simulink model "pmsm_vector_ctrl_osm_3_2021_06_21"  (R2020a)
settings: Solver=daessc  StartTime=0.0  StopTime=simlength  MaxStep=Ts/10
values from neighbouring files (symbols this model uses):
  dead_time = 0    [init_pmsm_2021_06_21.m]
  delayINV_modA = 0    [init_pmsm_2021_06_21.m]
  fPWM_INV = 8e3    (= 8000)    [init_pmsm_2021_06_21.m]
  Ibez = 450    [init_pmsm_2021_06_21.m]
  Jm = 1    [init_pmsm_2021_06_21.m]
  ki = 18    [init_pmsm_2021_06_21.m]
  kp = 2    [init_pmsm_2021_06_21.m]
  Ld = 1.7e-3    (= 0.0017)    [init_pmsm_2021_06_21.m]
  Lq = 4.3e-3    (= 0.0043)    [init_pmsm_2021_06_21.m]
  psi_m = 890/sqrt(3)/(3100/60*number_poles/2*2*pi)    [init_pmsm_2021_06_21.m]
  simlength = 5    [init_pmsm_2021_06_21.m]
  Tc = 1e-5    (= 1e-05)    [init_pmsm_2021_06_21.m]
  Ts = 1/10e3    (= 0.0001)    [init_pmsm_2021_06_21.m]
libraries: fl_lib x23, nesl_utility x22, ee_lib x6, flexshaft_lib x1, pmsm_uvw_lib x1
(part 2 of 2)

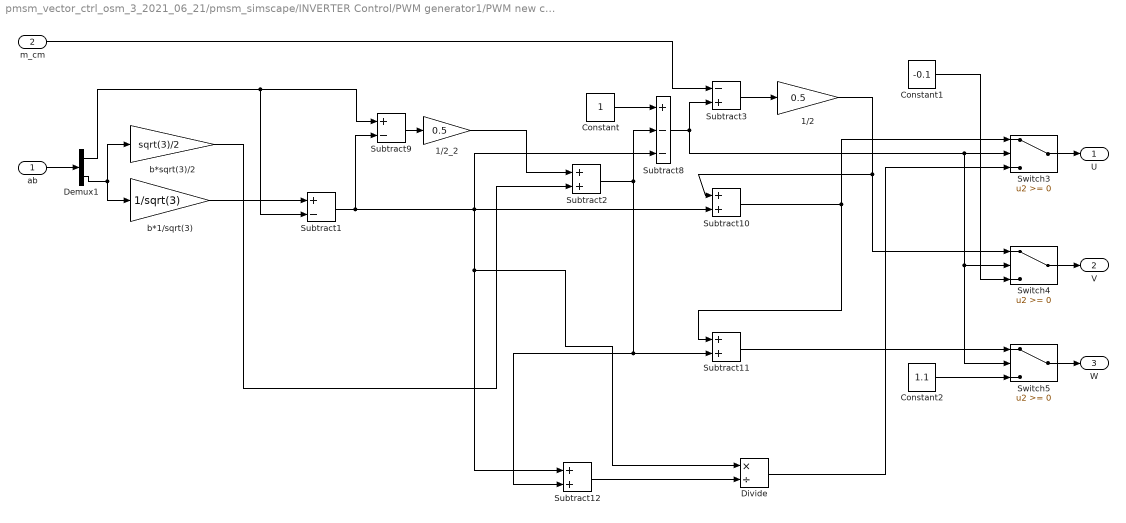
== system pmsm_vector_ctrl_osm_3_2021_06_21/pmsm_simscape/INVERTER Control/PWM generator1/PWM new cm modulation/Sector2 ==
  ab : Inport
  m_cm : Inport  Port=2
  1/2 : Gain  Gain=0.5
  1/2_2 : Gain  Gain=0.5
  Constant : Constant
  Constant1 : Constant  Value=-0.1
  Constant2 : Constant  Value=1.1
  Demux1 : Demux  Outputs=2
  Divide : Product  Inputs=*/
  Subtract1 : Sum  Inputs=+-
  Subtract{2,10..12} (4 alike) : Sum
  Subtract3 : Sum  Inputs=-+
  Subtract8 : Sum  Inputs=+--
  Subtract9 : Sum  Inputs=+-
  Switch3 : Switch
  Switch4 : Switch
  Switch5 : Switch
  b*1/sqrt(3) : Gain  Gain=1/sqrt(3)
  b*sqrt(3)/2 : Gain  Gain=sqrt(3)/2
  U : Outport
  V : Outport  Port=2
  W : Outport  Port=3
  wires:
  1/2/1 -> Switch4/1, Subtract10/1
  m_cm/1 -> Subtract3/1
  Subtract10/1 -> Subtract11/1, Switch3/1
  Constant2/1 -> Switch5/3
  Divide/1 -> Switch3/3
  Constant1/1 -> Switch4/3
  Subtract3/1 -> 1/2/1
  Subtract2/1 -> Subtract11/2, Subtract12/2, Subtract8/2
  b*sqrt(3)/2/1 -> Subtract2/2
  1/2_2/1 -> Subtract2/1
  Subtract9/1 -> 1/2_2/1
  Subtract1/1 -> Subtract9/2, Subtract8/3, Subtract10/2, Divide/1, Subtract12/1
  b*1/sqrt(3)/1 -> Subtract1/1
  Switch5/1 -> W/1
  Switch4/1 -> V/1
  Switch3/1 -> U/1
  ab/1 -> Demux1/1
  Subtract8/1 -> Switch5/2, Switch4/2, Switch3/2, Subtract3/2
  Constant/1 -> Subtract8/1
  Subtract11/1 -> Switch5/1
  Subtract12/1 -> Divide/2
  Demux1/1 -> Subtract1/2, Subtract9/1
  Demux1/2 -> b*sqrt(3)/2/1, b*1/sqrt(3)/1

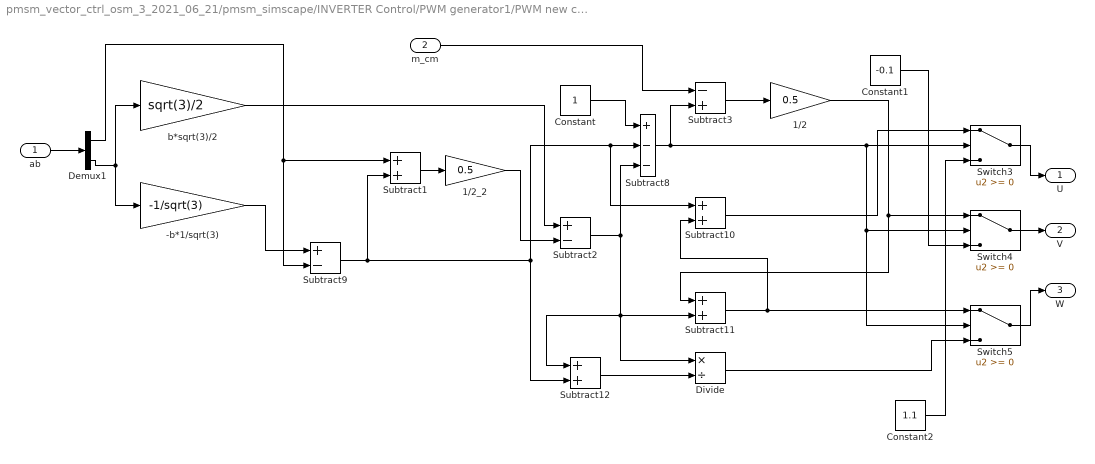
== system pmsm_vector_ctrl_osm_3_2021_06_21/pmsm_simscape/INVERTER Control/PWM generator1/PWM new cm modulation/Sector3 ==
  ab : Inport
  m_cm : Inport  Port=2
  -b*1/sqrt(3) : Gain  Gain=-1/sqrt(3)
  1/2 : Gain  Gain=0.5
  1/2_2 : Gain  Gain=0.5
  Constant : Constant
  Constant1 : Constant  Value=-0.1
  Constant2 : Constant  Value=1.1
  Demux1 : Demux  Outputs=2
  Divide : Product  Inputs=*/
  Subtract{1,10..12} (4 alike) : Sum
  Subtract2 : Sum  Inputs=+-
  Subtract3 : Sum  Inputs=-+
  Subtract8 : Sum  Inputs=+--
  Subtract9 : Sum  Inputs=+-
  Switch3 : Switch
  Switch4 : Switch
  Switch5 : Switch
  b*sqrt(3)/2 : Gain  Gain=sqrt(3)/2
  U : Outport
  V : Outport  Port=2
  W : Outport  Port=3
  wires:
  1/2/1 -> Switch4/1, Subtract11/1
  m_cm/1 -> Subtract3/1
  Constant1/1 -> Switch4/3
  Constant2/1 -> Switch3/3
  Divide/1 -> Switch5/3
  Subtract10/1 -> Switch3/1
  Subtract11/1 -> Subtract10/2, Switch5/1
  Subtract3/1 -> 1/2/1
  1/2_2/1 -> Subtract2/2
  Subtract1/1 -> 1/2_2/1
  b*sqrt(3)/2/1 -> Subtract2/1
  Subtract2/1 -> Subtract11/2, Divide/1, Subtract12/1, Subtract8/3
  Subtract9/1 -> Subtract12/2, Subtract8/2, Subtract10/1, Subtract1/2
  Demux1/1 -> Subtract9/2, Subtract1/1
  -b*1/sqrt(3)/1 -> Subtract9/1
  Demux1/2 -> -b*1/sqrt(3)/1, b*sqrt(3)/2/1
  Subtract12/1 -> Divide/2
  Constant/1 -> Subtract8/1
  Subtract8/1 -> Switch3/2, Switch4/2, Switch5/2, Subtract3/2
  ab/1 -> Demux1/1
  Switch3/1 -> U/1
  Switch4/1 -> V/1
  Switch5/1 -> W/1

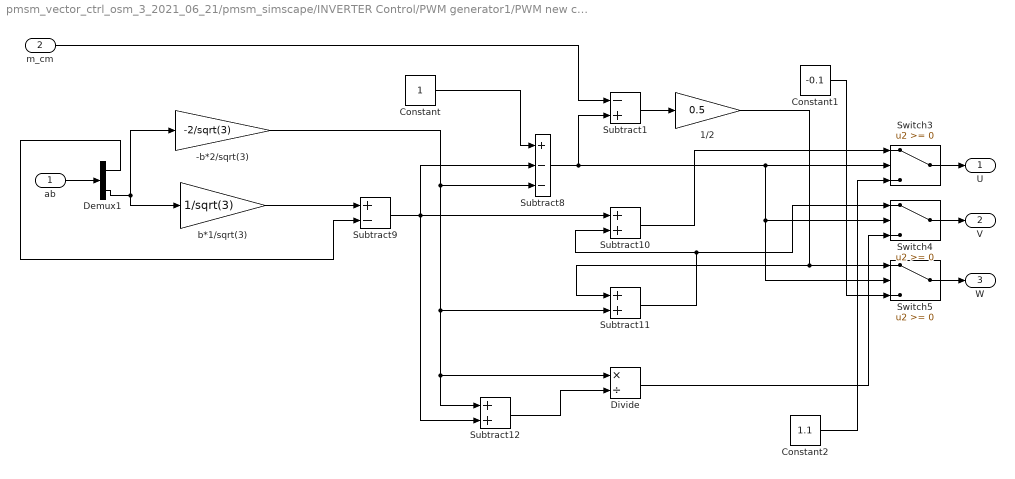
== system pmsm_vector_ctrl_osm_3_2021_06_21/pmsm_simscape/INVERTER Control/PWM generator1/PWM new cm modulation/Sector4 ==
  ab : Inport
  m_cm : Inport  Port=2
  -b*2/sqrt(3) : Gain  Gain=-2/sqrt(3)
  1/2 : Gain  Gain=0.5
  Constant : Constant
  Constant1 : Constant  Value=-0.1
  Constant2 : Constant  Value=1.1
  Demux1 : Demux  Outputs=2
  Divide : Product  Inputs=*/
  Subtract1 : Sum  Inputs=-+
  Subtract10 : Sum
  Subtract11 : Sum
  Subtract12 : Sum
  Subtract8 : Sum  Inputs=+--
  Subtract9 : Sum  Inputs=+-
  Switch3 : Switch
  Switch4 : Switch
  Switch5 : Switch
  b*1/sqrt(3) : Gain  Gain=1/sqrt(3)
  U : Outport
  V : Outport  Port=2
  W : Outport  Port=3
  wires:
  1/2/1 -> Switch5/1, Subtract11/1
  m_cm/1 -> Subtract1/1
  Constant1/1 -> Switch5/3
  Constant2/1 -> Switch3/3
  Divide/1 -> Switch4/3
  Subtract11/1 -> Switch4/1, Subtract10/2
  Subtract10/1 -> Switch3/1
  Subtract1/1 -> 1/2/1
  -b*2/sqrt(3)/1 -> Subtract8/3, Subtract11/2, Divide/1, Subtract12/1
  Subtract9/1 -> Subtract12/2, Subtract10/1, Subtract8/2
  Demux1/1 -> Subtract9/2
  b*1/sqrt(3)/1 -> Subtract9/1
  Switch5/1 -> W/1
  Switch4/1 -> V/1
  Switch3/1 -> U/1
  ab/1 -> Demux1/1
  Subtract8/1 -> Switch5/2, Switch4/2, Switch3/2, Subtract1/2
  Constant/1 -> Subtract8/1
  Subtract12/1 -> Divide/2
  Demux1/2 -> b*1/sqrt(3)/1, -b*2/sqrt(3)/1

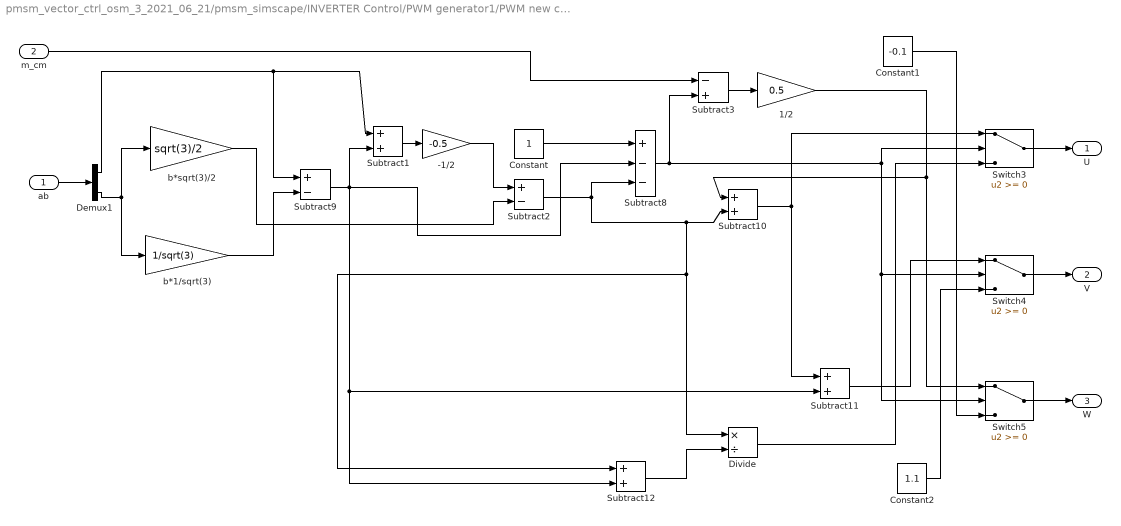
== system pmsm_vector_ctrl_osm_3_2021_06_21/pmsm_simscape/INVERTER Control/PWM generator1/PWM new cm modulation/Sector5 ==
  ab : Inport
  m_cm : Inport  Port=2
  -1/2 : Gain  Gain=-0.5
  1/2 : Gain  Gain=0.5
  Constant : Constant
  Constant1 : Constant  Value=-0.1
  Constant2 : Constant  Value=1.1
  Demux1 : Demux  Outputs=2
  Divide : Product  Inputs=*/
  Subtract{1,10..12} (4 alike) : Sum
  Subtract2 : Sum  Inputs=+-
  Subtract3 : Sum  Inputs=-+
  Subtract8 : Sum  Inputs=+--
  Subtract9 : Sum  Inputs=+-
  Switch3 : Switch
  Switch4 : Switch
  Switch5 : Switch
  b*1/sqrt(3) : Gain  Gain=1/sqrt(3)
  b*sqrt(3)/2 : Gain  Gain=sqrt(3)/2
  U : Outport
  V : Outport  Port=2
  W : Outport  Port=3
  wires:
  1/2/1 -> Switch5/1, Subtract10/1
  m_cm/1 -> Subtract3/1
  Constant2/1 -> Switch4/3
  Divide/1 -> Switch3/3
  Subtract11/1 -> Switch4/1
  Subtract10/1 -> Subtract11/1, Switch3/1
  Constant1/1 -> Switch5/3
  Subtract3/1 -> 1/2/1
  Subtract2/1 -> Subtract8/3, Divide/1, Subtract12/1, Subtract10/2
  b*sqrt(3)/2/1 -> Subtract2/2
  -1/2/1 -> Subtract2/1
  Subtract1/1 -> -1/2/1
  Subtract9/1 -> Subtract11/2, Subtract12/2, Subtract8/2, Subtract1/2
  Demux1/2 -> b*1/sqrt(3)/1, b*sqrt(3)/2/1
  Demux1/1 -> Subtract1/1, Subtract9/1
  Subtract12/1 -> Divide/2
  b*1/sqrt(3)/1 -> Subtract9/2
  Constant/1 -> Subtract8/1
  Subtract8/1 -> Switch3/2, Switch4/2, Switch5/2, Subtract3/2
  ab/1 -> Demux1/1
  Switch3/1 -> U/1
  Switch4/1 -> V/1
  Switch5/1 -> W/1

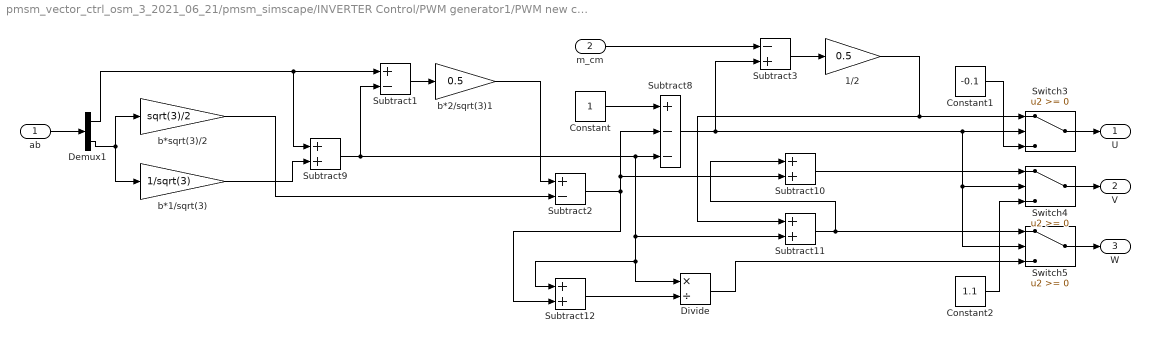
== system pmsm_vector_ctrl_osm_3_2021_06_21/pmsm_simscape/INVERTER Control/PWM generator1/PWM new cm modulation/Sector6 ==
  ab : Inport
  m_cm : Inport  Port=2
  1/2 : Gain  Gain=0.5
  Constant : Constant
  Constant1 : Constant  Value=-0.1
  Constant2 : Constant  Value=1.1
  Demux1 : Demux  Outputs=2
  Divide : Product  Inputs=*/
  Subtract1 : Sum  Inputs=+-
  Subtract{9..12} (4 alike) : Sum
  Subtract2 : Sum  Inputs=+-
  Subtract3 : Sum  Inputs=-+
  Subtract8 : Sum  Inputs=+--
  Switch3 : Switch
  Switch4 : Switch
  Switch5 : Switch
  b*1/sqrt(3) : Gain  Gain=1/sqrt(3)
  b*2/sqrt(3)1 : Gain  Gain=0.5
  b*sqrt(3)/2 : Gain  Gain=sqrt(3)/2
  U : Outport
  V : Outport  Port=2
  W : Outport  Port=3
  wires:
  1/2/1 -> Switch3/1, Subtract11/1
  m_cm/1 -> Subtract3/1
  Constant2/1 -> Switch4/3
  Divide/1 -> Switch5/3
  Subtract2/1 -> Subtract12/2, Subtract10/2, Subtract8/2
  b*sqrt(3)/2/1 -> Subtract2/2
  b*2/sqrt(3)1/1 -> Subtract2/1
  Subtract1/1 -> b*2/sqrt(3)1/1
  Demux1/2 -> b*1/sqrt(3)/1, b*sqrt(3)/2/1
  Demux1/1 -> Subtract1/1, Subtract9/1
  Subtract12/1 -> Divide/2
  Constant1/1 -> Switch3/3
  Subtract11/1 -> Subtract10/1, Switch5/1
  Subtract10/1 -> Switch4/1
  Subtract3/1 -> 1/2/1
  b*1/sqrt(3)/1 -> Subtract9/2
  Subtract9/1 -> Subtract8/3, Subtract11/2, Divide/1, Subtract12/1, Subtract1/2
  Constant/1 -> Subtract8/1
  Subtract8/1 -> Switch3/2, Switch4/2, Switch5/2, Subtract3/2
  ab/1 -> Demux1/1
  Switch3/1 -> U/1
  Switch4/1 -> V/1
  Switch5/1 -> W/1

== system pmsm_vector_ctrl_osm_3_2021_06_21/pmsm_simscape/INVERTER Control/PWM generator1/PWM new cm modulation/Shifted_triangle down ==
  Constant1 : Constant  Value=1/2-dead_time*fPWM_INV
  Gain1 : Gain  Gain=1/(pi)
  Sine Wave1 : Sin  Frequency=fPWM_INV*2*pi  Phase=-pi/2+delayINV_modA
  Subtract12 : Sum
  Trigonometric Function2 : Trigonometry  Operator=asin
  Out1 : Outport
  wires:
  Subtract12/1 -> Out1/1
  Gain1/1 -> Subtract12/1
  Constant1/1 -> Subtract12/2
  Sine Wave1/1 -> Trigonometric Function2/1
  Trigonometric Function2/1 -> Gain1/1

== system pmsm_vector_ctrl_osm_3_2021_06_21/pmsm_simscape/INVERTER Control/PWM generator1/PWM new cm modulation/Shifted_triangle up ==
  Constant1 : Constant  Value=1/2+dead_time*fPWM_INV
  Gain1 : Gain  Gain=1/(pi)
  Sine Wave1 : Sin  Frequency=fPWM_INV*2*pi  Phase=-pi/2+delayINV_modA
  Subtract12 : Sum
  Trigonometric Function2 : Trigonometry  Operator=asin
  Out1 : Outport
  wires:
  Trigonometric Function2/1 -> Gain1/1
  Sine Wave1/1 -> Trigonometric Function2/1
  Constant1/1 -> Subtract12/2
  Gain1/1 -> Subtract12/1
  Subtract12/1 -> Out1/1

== matlab function pmsm_vector_ctrl_osm_3_2021_06_21/mtpa ==
  data: Ld input; Lq input; psi_m input; iq input; id output; Ibez input
function id  = mtpa(Ld,Lq,psi_m,iq,Ibez)



id = (psi_m/2/(Lq-Ld)-sqrt(psi_m^2/4/(Lq-Ld)^2+(iq*Ibez)^2))/Ibez;
end
